simulink model "sm_car_testrig_bus_VehBusChassisWhlFL"  (R2019a)
settings: Solver=VariableStepAuto  StartTime=0.0  StopTime=10.0  RelTol=1e-3
libraries: sm_car_lib x3, sm_lib x2, Tire_Models x1, nesl_utility x1
Description:
  | Copyright 2020 The MathWorks, Inc.
settings Model: Creator=smiller  LastModifiedBy=smiller
settings DataIOCC: ReturnWorkspaceOutputs=off
settings DebuggingCC: ArithmeticOperatorsInVariantConditions=warning
settings DiagnosticsConfigSet: SimMechanicsConflictingReferenceFrames=none  SimMechanicsRigidlyBoundBlock=none
settings ExplorerConfigSet: SimMechanicsOpenEditorOnUpdate=off

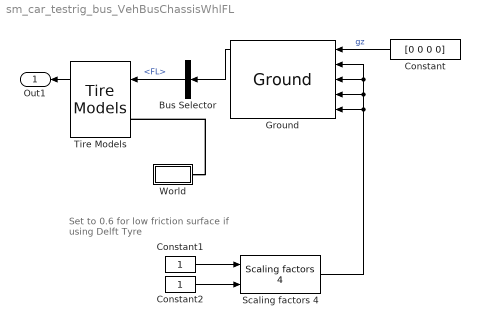
== system sm_car_testrig_bus_VehBusChassisWhlFL ==
  note: Set to 0.6 for low friction
      | surface if using Delft Tyre
  Bus Selector : BusSelector  OutputSignals=FL
  Constant : Constant  Value=[0 0 0 0]
  Constant1 : Constant
  Constant2 : Constant
  Ground : sm_car_lib/Tires/Ground  SystemSampleTime=-1
  Scaling factors 4 : sm_car_lib/Tires/Scaling factors 4  LKX=1  LKY=1  LKYC=1  LTR=1  LKZC=1
  Tire Models : Tire_Models/Tire Models  Tag=PublishSubsystem  VariantControl=Variant1  popup_leftRight=Right  tir_index=1  Tire=Vehicle.Chassis.TyreF  VariantLabel=Vehicle.Chassis.TyreF.class.Value  InitTriggerDropdown=1
      settings: AttributesFormatString=%<ActiveVariant>
  World : Subsystem
      mask Display: disp('Wld')
  Out1 : Outport  OutDataTypeStr=Bus: VehicleChassisWhlFLBusDef
  wires:
  Tire Models/1 -> Out1/1
  Constant/1 -> Ground/1  "gz"
  Constant1/1 -> Scaling factors 4/1
  Scaling factors 4/1 -> Ground/5, Ground/4, Ground/2, Ground/3
  Ground/1 -> Bus Selector/1
  Constant2/1 -> Scaling factors 4/2
  Bus Selector/1 -> Tire Models/1  "<FL>"
  connections:
  World/RConn1 -- Tire Models/LConn1

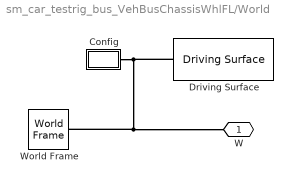
== system sm_car_testrig_bus_VehBusChassisWhlFL/World ==
  Config : Subsystem
  Driving Surface : sm_car_lib/Environment/Driving Surface  LabelModeActiveChoice=Floor_Grid
  World Frame : sm_lib/Frames and Transforms/World Frame
  W : PMIOPort  Side=Right
  connections:
  Config/RConn1 -- Driving Surface/RConn1 -- World Frame/RConn1 -- W/RConn1

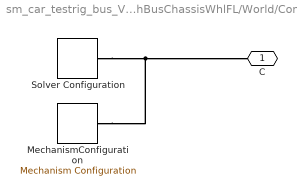
== system sm_car_testrig_bus_VehBusChassisWhlFL/World/Config ==
  MechanismConfiguration : sm_lib/Utilities/Mechanism Configuration  UniformGravity=Constant  GravityVector=[0 0 -9.80665]  GravityUnits=m/s^2  LinearizationDelta=0.001
  Solver Configuration : nesl_utility/Solver Configuration  PhysicalDomain=network_engine_domain  SubClassName=solver  LeftPortType=input  RightPortType=generic  Tones=[]  Harmonics=[]  SimulateNoise=off  Profile=off  UseLocalSampling=off  EnableSwitchedLinearOptims=on  FrequencyDomain=off  UseCCode=off  RelTol=0.001  AbsTol=1e-06  MinStep=1e-09  ToWorkspace=off  RevertToSquareIcSolve=off  NumHomotopyIterations=100  PhasorMode=off  PhasorModeNumHarmonics=1  DoDC=off  ResidualTolerance=1e-9  UseLocalSolver=off  LocalSolverChoice=NE_BACKWARD_EULER_ADVANCER  LocalSolverSampleTime=0.00025*4  DoFixedCost=off  MaxNonlinIter=3  MaxModeIter=2  LinearAlgebra=Sparse  EquationFormulation=NE_TIME_EF  DelaysMemoryBudget=1024  AutomaticFiltering=on  FilteringTimeConstant=0.001  PartitionStorageMethod=AS_NEEDED  PartitionMemoryBudget=1024  PartitionMethod=FAST
  C : PMIOPort  Side=Right
  connections:
  Solver Configuration/RConn1 -- C/RConn1 -- MechanismConfiguration/RConn1
